simulink model "SalientPolePMSM"  (R2020b)
settings: Solver=VariableStepAuto  StartTime=0  StopTime=1  MaxStep=1e-4  RelTol=1e-4
values from neighbouring files (symbols this model uses):
  Bgain = 1    [DataSalientPolePMSM-DESKTOP-IINSHMA.m]    (also in DataSalientPolePMSM.m)
  Gcc_1ord = 1/(s/bandwidth(Gcc) + 1)    [DataSalientPolePMSM-DESKTOP-IINSHMA.m]    (also in DataSalientPolePMSM.m)
  lamdVec = mot.Ld*idVec+mot.lammg    [DataSalientPolePMSM-DESKTOP-IINSHMA.m]    (also in DataSalientPolePMSM.m)
  lamqVec = mot.Lq*iqVec    [DataSalientPolePMSM-DESKTOP-IINSHMA.m]    (also in DataSalientPolePMSM.m)
  TAB0_abc = Tabc_AB0^-1    [DataSalientPolePMSM-DESKTOP-IINSHMA.m]    (also in DataSalientPolePMSM.m)
  Tabc_AB0 = 2/3.*[     1       -1/2       -1/2 ... (first row only)    [DataSalientPolePMSM-DESKTOP-IINSHMA.m]    (also in DataSalientPolePMSM.m)
  Talphabeta_abc = Tabc_alphabeta^(-1)    [DataSalientPolePMSM-DESKTOP-IINSHMA.m]    (also in DataSalientPolePMSM.m)
undefined symbols (not defined in the file or in its folder): DiscIntNeverNeededParam, dqpll, inv, kid, kpd, magnitude, meas, mot, Obs, PI, stconv
libraries: simulink x53, pid_lib x3, powerlib x2, eeBldcCommutationLogic x1, electricdrivelib x1
(part 1 of 7)
settings Model: Creator=checc  LastModifiedBy=giuli
settings DataIOCC: SaveFormat=StructureWithTime

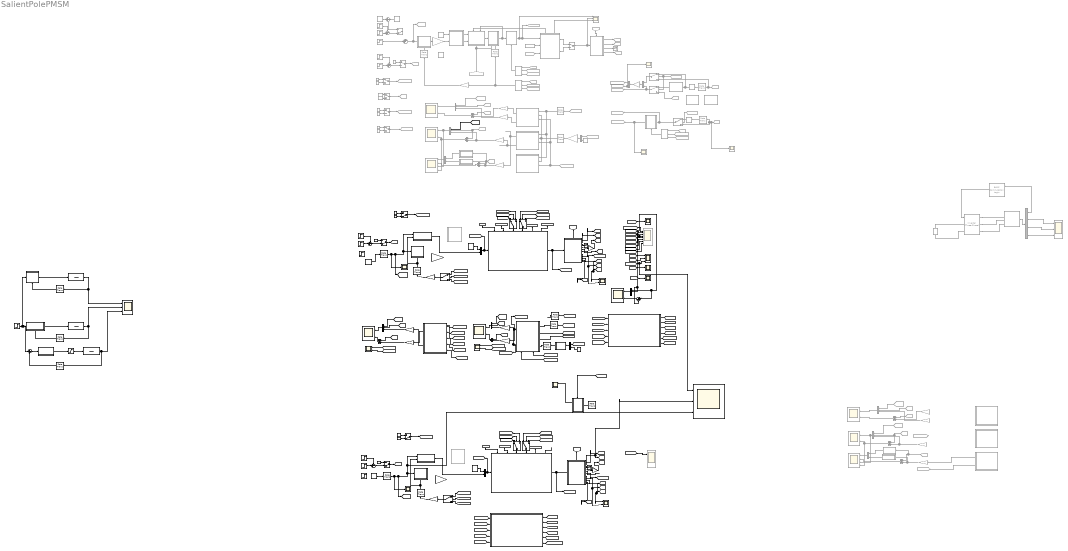
== system SalientPolePMSM ==
  note: Fuzzy Test
  note: COMMANDS
  note: GIULIO SAVIAN MODEL
  note: RICCARDO CHECHIN MODEL
  note: SIMSCAPE MODEL
  note: FEEDBACK
  note: PMSM MOTOR
  note: FIELD ORIENTED CONTROL ALGORITHM
  note: SCOPE
  note: CONTROL PANEL
  note: SENSORLESS ALGORITHM
  note: MTPA strategy
  note: FEEDBACK CHAIN
  note: INPUTS
  note: Consider the inverter
      | nonidealities or not
  note: INPUTS
  note: OUTPUTS
  note: MTPA strategy
  note: SENSORLESS ALGORITHM alpha beta axis
  note: SENSORLESS ALGORITHM dq axis (NON FUNZIONANTE)
  note: COMMANDS
  note: INPUTS
  note: FIELD ORIENTED CONTROL ALGORITHM
  note: MTPA strategy
  note: PMSM MOTOR
  " 1" : MATLAB Function  TreatAsAtomicUnit=on
  AC Voltage Source : powerlib/Electrical Sources/AC Voltage Source  Commented=on  Amplitude=100  Phase=0  Frequency=60  SampleTime=0  Measurements=None  BusType=swing  Pref=10e3  Qref=0  Qmin=-inf  Qmax=+inf
  Avarage Derivative : MATLAB Function  Commented=on  TreatAsAtomicUnit=on
  BLDC Commutation Logic : eeBldcCommutationLogic/BLDC Commutation Logic  Commented=on  Ts=-1
      settings: SourceProductBaseCode=PS
  Clarke + Park 5 : Subsystem
      settings: PortSchema="{\"entries\":[{\"content\":{\"sides\":[{\"content\":{\"connectorIds\":[\"In1\"]},\"type\":\"ConnectorPlacement.EquallySpacedRectSide\",\"uuid\":\"e456cd5a-7662-4e0b-a6c7-27ed01a0cde8\"},{\"content\":{\"connectorIds\":[\"Out1\",\"Out2\"],\"side\":\"RIGHT\"},\"type\":\"ConnectorPlacement.EquallySpacedRectSide\",\"uuid\":\"028e266b-db3d-4fa0-9acb-55f4e679375c\"},{\"content\":{\"connectorIds\":[],\"side\":\"TOP\"},\"type\":\"ConnectorPlacement.EquallySpacedRectSide\",\"uuid\":\"fc8407b0-ab5c-4984-8f89-848ec890a8d5\"},{\"content\":{\"connectorIds\":[\"In2\"],\"side\":\"BOTTOM\"},\"type\":\"ConnectorPlacement.EquallySpacedRectSide\",\"uuid\":\"5b71beec-2170-4cb0-81b8-756f92b052d7\"},{\"content\":{\"connectorIds\":[],\"side\":\"HIDDEN\"},\"type\":\"ConnectorPlacement.EquallySpacedRectSide\",\"uuid\":\"110705d2-59f3-422e-b935-78b651f69ef1\"}]},\"type\":\"ConnectorPlacement.EquallySpacedConnector\",\"uuid\":\"4a76e66d-c848-4e9c-8e50-4d720647e920\"}],\"packageUris\":[\"http://schema.mathworks.com/mf0/Connector/R2020b\"],\"version\":\"1.0\"}"
  Constant{,7,9,13} (4 alike) : Constant  Commented=on
  Constant{1,3,8,10..11} (5 alike) : Constant  Commented=on  Value=0
  Constant{5..6,12,14..15,17,21} (7 alike) : Constant  Value=0
  Constant16 : Constant
  Constant2 : Constant  Commented=on  Value=2
  Constant22 : Constant
  Constant4 : Constant  Commented=on  Value=inv.Ubus
  Control 0- Sensorless 1-Sensor : ManualSwitch  CurrentSetting=0
  Control 0- Sensorless 1-Sensor1 : ManualSwitch  CurrentSetting=0
  DER+IIR_Butterworth : MATLAB Function  Commented=on  TreatAsAtomicUnit=on
  DT SENSORLESS ALGORITHM AB : Subsystem
  DT SENSORLESS ALGORITHM DQ : Subsystem
      settings: PortSchema="{\"entries\":[{\"content\":{\"sides\":[{\"content\":{\"connectorIds\":[\"In1\",\"In2\",\"In3\",\"In4\"]},\"type\":\"ConnectorPlacement.EquallySpacedRectSide\",\"uuid\":\"b3c8a319-13c6-48fe-86bb-1433f6356212\"},{\"content\":{\"connectorIds\":[\"Out1\",\"Out2\"],\"side\":\"RIGHT\"},\"type\":\"ConnectorPlacement.EquallySpacedRectSide\",\"uuid\":\"9e7987ae-9f82-46ba-9b9e-b4e3c3a64e56\"},{\"content\":{\"connectorIds\":[],\"side\":\"TOP\"},\"type\":\"ConnectorPlacement.EquallySpacedRectSide\",\"uuid\":\"daf6aa39-0b26-4777-9886-9f84f51f9a28\"},{\"content\":{\"connectorIds\":[\"In5\",\"In6\"],\"side\":\"BOTTOM\"},\"type\":\"ConnectorPlacement.EquallySpacedRectSide\",\"uuid\":\"08005c1e-9a10-4744-b3a8-492e89e20f7c\"},{\"content\":{\"connectorIds\":[],\"side\":\"HIDDEN\"},\"type\":\"ConnectorPlacement.EquallySpacedRectSide\",\"uuid\":\"78ab3349-e4d4-4e96-9309-6e60ebf678be\"}]},\"type\":\"ConnectorPlacement.EquallySpacedConnector\",\"uuid\":\"6a0093e8-1b7a-497c-85fe-0bb07724db39\"}],\"packageUris\":[\"http://schema.mathworks.com/mf0/Connector/R2020b\"],\"version\":\"1.0\"}"
  Decoupling : Subsystem  Commented=on
      settings: PortSchema="{\"entries\":[{\"content\":{\"sides\":[{\"content\":{\"connectorIds\":[\"In1\"]},\"type\":\"ConnectorPlacement.EquallySpacedRectSide\",\"uuid\":\"366d4760-99ea-4839-93ce-cd028ffff2ed\"},{\"content\":{\"connectorIds\":[\"Out1\"],\"side\":\"RIGHT\"},\"type\":\"ConnectorPlacement.EquallySpacedRectSide\",\"uuid\":\"ffb80cd0-5569-4ccd-9b8e-dc37fbe2d6f7\"},{\"content\":{\"connectorIds\":[],\"side\":\"TOP\"},\"type\":\"ConnectorPlacement.EquallySpacedRectSide\",\"uuid\":\"2e02478e-0c74-4c41-9c3e-8c0e6bb6923b\"},{\"content\":{\"connectorIds\":[\"In2\",\"In3\"],\"side\":\"BOTTOM\"},\"type\":\"ConnectorPlacement.EquallySpacedRectSide\",\"uuid\":\"0c356034-c9d0-432b-942d-38470146113e\"}]},\"type\":\"ConnectorPlacement.EquallySpacedConnector\",\"uuid\":\"999d36d2-be3d-4c0f-9dc8-4c30e8aa3320\"}],\"packageUris\":[\"http://schema.mathworks.com/mf0/Connector/19700101\"],\"version\":\"1.0\"}"
  Demux : Demux  Commented=on  Outputs=2
  Demux1 : Demux  Commented=on
  Discrete SS ALGORITHM : Subsystem  Commented=on
  Discrete SS ALGORITHM1 : Subsystem  Commented=on
  FEEDBACK1 : Scope  Commented=on  NumInputPorts=8
  FEEDBACK2 : Scope  Commented=on  NumInputPorts=8
  FOC1 : Subsystem
      settings: PortSchema="{\"entries\":[{\"content\":{\"sides\":[{\"content\":{\"connectorIds\":[\"In1\"]},\"type\":\"ConnectorPlacement.EquallySpacedRectSide\",\"uuid\":\"8f808d96-7d84-4ca2-a92f-a817aa87351b\"},{\"content\":{\"connectorIds\":[\"Out1\"],\"side\":\"RIGHT\"},\"type\":\"ConnectorPlacement.EquallySpacedRectSide\",\"uuid\":\"5a731029-8147-494c-b637-5944669b2a42\"},{\"content\":{\"connectorIds\":[\"In2\",\"In3\",\"In4\",\"In5\",\"Out2\",\"Out3\"],\"side\":\"TOP\"},\"type\":\"ConnectorPlacement.EquallySpacedRectSide\",\"uuid\":\"612a65e4-5a0a-4716-ba74-ea18628a9a43\"},{\"content\":{\"connectorIds\":[],\"side\":\"HIDDEN\"},\"type\":\"ConnectorPlacement.EquallySpacedRectSide\",\"uuid\":\"5c37c74d-a0a6-4de5-9c93-6ea2c3953579\"}]},\"type\":\"ConnectorPlacement.EquallySpacedConnector\",\"uuid\":\"f471e1e3-c38d-4067-8334-0ee03542d9ee\"}],\"packageUris\":[\"http://schema.mathworks.com/mf0/Connector/R2020b\"],\"version\":\"1.0\"}"
  FOC2 : Subsystem
      settings: PortSchema="{\"entries\":[{\"content\":{\"sides\":[{\"content\":{\"connectorIds\":[\"In1\"]},\"type\":\"ConnectorPlacement.EquallySpacedRectSide\",\"uuid\":\"8f808d96-7d84-4ca2-a92f-a817aa87351b\"},{\"content\":{\"connectorIds\":[\"Out1\"],\"side\":\"RIGHT\"},\"type\":\"ConnectorPlacement.EquallySpacedRectSide\",\"uuid\":\"5a731029-8147-494c-b637-5944669b2a42\"},{\"content\":{\"connectorIds\":[\"In2\",\"In3\",\"In4\",\"In5\",\"Out2\",\"Out3\"],\"side\":\"TOP\"},\"type\":\"ConnectorPlacement.EquallySpacedRectSide\",\"uuid\":\"612a65e4-5a0a-4716-ba74-ea18628a9a43\"},{\"content\":{\"connectorIds\":[],\"side\":\"HIDDEN\"},\"type\":\"ConnectorPlacement.EquallySpacedRectSide\",\"uuid\":\"5c37c74d-a0a6-4de5-9c93-6ea2c3953579\"}]},\"type\":\"ConnectorPlacement.EquallySpacedConnector\",\"uuid\":\"f471e1e3-c38d-4067-8334-0ee03542d9ee\"}],\"packageUris\":[\"http://schema.mathworks.com/mf0/Connector/R2020b\"],\"version\":\"1.0\"}"
  FOC_out1 : Scope
  FeedBack: 1-MEASURE 2-SENSORLESS : ManualSwitch  Commented=on
  Feedback1 : Subsystem
  Feedback2 : Subsystem
  From : From  Commented=on  GotoTag=IABC
  From1 : From  Commented=on  GotoTag=THME_MEAS
  From10 : From  Commented=on  GotoTag=TAUL
  From{11,13,27..28,35} (5 alike) : From  Commented=on  GotoTag=THM
  From{5,14,25,29,33} (5 alike) : From  Commented=on  GotoTag=WM
  From15 : From  Commented=on  GotoTag=ON_MEAS
  From16 : From  Commented=on  GotoTag=ON_APPROX
  From17 : From  Commented=on  GotoTag=FEED
  From18 : From  Commented=on  GotoTag=WME_MEAS
  From19 : From  Commented=on  GotoTag=FEED
  From20 : From  Commented=on  GotoTag=WME_EST
  From21 : From  Commented=on  GotoTag=THME_MEAS
  From22 : From  Commented=on  GotoTag=FEED
  From23 : From  Commented=on  GotoTag=THME_EST
  From26 : From  Commented=on  GotoTag=W_REF
  From3 : From  Commented=on  GotoTag=IDQ_MEAS
  From31 : From  Commented=on  GotoTag=W_REF
  From34 : From  Commented=on  GotoTag=W_REF
  From4 : From  Commented=on  GotoTag=IABC
  From6 : From  Commented=on  GotoTag=UAB_REF
  From7 : From  Commented=on  GotoTag=THME_EST
  From8 : From  Commented=on  GotoTag=ON_MEAS
  From9 : From  Commented=on  GotoTag=IABC_MEAS
  Fuzzy PI : Subsystem
  Fuzzy PI1 : Subsystem
      settings: PortSchema="{\"entries\":[{\"content\":{\"sides\":[{\"content\":{\"connectorIds\":[\"In1\"]},\"type\":\"ConnectorPlacement.EquallySpacedRectSide\",\"uuid\":\"97881aea-ae0e-45c3-b7bb-3f05d1abc06d\"},{\"content\":{\"connectorIds\":[\"Out1\"],\"side\":\"RIGHT\"},\"type\":\"ConnectorPlacement.EquallySpacedRectSide\",\"uuid\":\"622239dd-e339-479b-bebf-0984d9e159b9\"},{\"content\":{\"connectorIds\":[],\"side\":\"TOP\"},\"type\":\"ConnectorPlacement.EquallySpacedRectSide\",\"uuid\":\"04f8ad64-72f6-4003-b853-88924601f787\"},{\"content\":{\"connectorIds\":[\"In2\"],\"side\":\"BOTTOM\"},\"type\":\"ConnectorPlacement.EquallySpacedRectSide\",\"uuid\":\"da7a61ed-22a9-4131-8461-57923f50db6b\"},{\"content\":{\"connectorIds\":[],\"side\":\"HIDDEN\"},\"type\":\"ConnectorPlacement.EquallySpacedRectSide\",\"uuid\":\"98b26063-fb72-4532-826e-e0a43804adb7\"}]},\"type\":\"ConnectorPlacement.EquallySpacedConnector\",\"uuid\":\"af8a33e1-8440-4bbf-a2b8-49fd6263fc38\"}],\"packageUris\":[\"http://schema.mathworks.com/mf0/Connector/R2020b\"],\"version\":\"1.0\"}"
  Fuzzy PI2 : Subsystem
  Gain : Gain  Commented=on  Gain=1/mot.kTau
  Gain{1,3..5,7,11..14} (9 alike) : Gain  Commented=on  Gain=1/mot.p
  Gain10 : Gain  Gain=Bgain
  Gain15 : Gain  Gain=Bgain
  Gain{9,16..17,19..21} (6 alike) : Gain  Gain=1/mot.p
  Gain18 : Gain  Gain=1/mot.kTau
  Gain2 : Gain  Commented=on  Gain=mot.p
  Gain6 : Gain  Gain=1/mot.kTau
  Gain8 : Gain  Commented=on  Gain=TAB0_abc  Multiplication=Matrix(K*u) (u vector)
  Goto : Goto  Commented=on  GotoTag=IABC
  Goto1 : Goto  Commented=on  GotoTag=THM
  Goto10 : Goto  Commented=on  GotoTag=WM
  Goto11 : Goto  Commented=on  GotoTag=FEED
  Goto12 : Goto  Commented=on  GotoTag=ON_MEAS
  Goto13 : Goto  Commented=on  GotoTag=IABC_MEAS
  Goto14 : Goto  Commented=on  GotoTag=ON_APPROX
  Goto15 : Goto  Commented=on  GotoTag=ADD_INT
  Goto16 : Goto  Commented=on  GotoTag=W_REF
  Goto18 : Goto  Commented=on  GotoTag=THME_EST
  Goto19 : Goto  Commented=on  GotoTag=WME_EST
  Goto2 : Goto  Commented=on  GotoTag=UAB_REF
  Goto3 : Goto  Commented=on  GotoTag=IDQ_MEAS
  Goto5 : Goto  Commented=on  GotoTag=WM_MEAS
  Goto6 : Goto  Commented=on  GotoTag=TAUL
  Goto7 : Goto  Commented=on  GotoTag=THME_MEAS
  Goto8 : Goto  Commented=on  GotoTag=WME_MEAS
  HPF FIR : MATLAB Function  Commented=on  TreatAsAtomicUnit=on
  INPUTS1 : Scope
  INVERTER : Subsystem  Commented=on
      settings: PortSchema="{\"entries\":[{\"content\":{\"sides\":[{\"content\":{\"connectorIds\":[\"In1\",\"In2\",\"In3\"]},\"type\":\"ConnectorPlacement.EquallySpacedRectSide\",\"uuid\":\"79c77d12-022f-42ce-98d0-f3ead9d04a95\"},{\"content\":{\"connectorIds\":[\"Out1\",\"Out2\"],\"side\":\"RIGHT\"},\"type\":\"ConnectorPlacement.EquallySpacedRectSide\",\"uuid\":\"afd498dc-a72a-45ee-96a4-44488bf591ce\"},{\"content\":{\"connectorIds\":[\"Out3\",\"Out4\"],\"side\":\"TOP\"},\"type\":\"ConnectorPlacement.EquallySpacedRectSide\",\"uuid\":\"f8f8ad46-d0da-4286-941c-855cc15ed51d\"}]},\"type\":\"ConnectorPlacement.EquallySpacedConnector\",\"uuid\":\"436ef73d-4718-409e-82fb-57ff2ccd93cf\"}],\"packageUris\":[\"http://schema.mathworks.com/mf0/Connector/R2020b\"],\"version\":\"1.0\"}"
  Inverter (Three-Phase) : electricdrivelib/Fundamental Drive Blocks/Inverter (Three-Phase)  Commented=on  LabelModeActiveChoice=Detailed  detailLevel=Detailed  driveType=Field-oriented control  Ts=2e-6  SnubberResistance=10e3  SnubberCapacitance=inf  Device=IGBT / Diodes  Ron=1e-3  ForwardVoltages=[1.2,1.2]  GTOparameters=[1e-6,2e-6]  IGBTparameters=[1e-6,2e-6]  Measurements=All voltages and currents  converterType=Inverter  SourceFrequency=60  ReferenceFrame=Rotor  dqInductances=[8.5e-3,8.5e-3]  Inductance=8.5e-3  Ls=0  Resistance=0.2  Flux=0.175  Stator_sm=[2.01e-3,4.289e-4,4.477e-3,1.354e-3]  Stator_im=[14.85e-3,0.3027e-3]  Rotor=[9.295e-3,0.3027e-3]  Lm=10.46e-3  p=4
      settings: AttributesFormatString=%<BlockChoice>  SourceProductBaseCode=PS
  MATLAB Function : MATLAB Function  Commented=on  TreatAsAtomicUnit=on
  MATLAB Function1 : MATLAB Function  Commented=on  TreatAsAtomicUnit=on
  MATLAB Function2 : MATLAB Function  Commented=on  TreatAsAtomicUnit=on
  MATLAB Function3 : MATLAB Function  Commented=on  TreatAsAtomicUnit=on
  MATLAB Function4 : MATLAB Function  Commented=on  TreatAsAtomicUnit=on
  MATLAB Function5 : MATLAB Function  Commented=on  TreatAsAtomicUnit=on
  MATLAB Function6 : MATLAB Function  Commented=on  TreatAsAtomicUnit=on
  MOTOR2 : Scope  NumInputPorts=3
  MTPA 1- id=0 0- id!=0 : Constant  Commented=on  Value=0  SampleTime=PI.vel.Ts
  MTPA 1- id=0 0- id!=1 : Constant  Commented=on  Value=0.5  SampleTime=PI.vel.Ts
  Manual Switch : ManualSwitch  Commented=on
  Measures: 0-Ideal 1-Real : ManualSwitch  Commented=on
  Multiport Switch1 : MultiPortSwitch  Commented=on  Inputs=2
  Multiport Switch2 : MultiPortSwitch  Commented=on  Inputs=2
  Multiport Switch4 : MultiPortSwitch  Commented=on  Inputs=2
  Mux{,2,4,9} (4 alike) : Mux  Commented=on  Inputs=2
  Mux1 : Mux  Inputs=2
  Mux{3,5,8,10} (4 alike) : Mux  Commented=on  Inputs=3
  Mux11 : Mux  Inputs=3
  Mux12 : Mux  Inputs=3
  Mux13 : Mux  Inputs=3
  Mux6 : Mux  Inputs=2
  Mux7 : Mux  Inputs=2
  PI_curr : Subsystem  Commented=on
      settings: PortSchema="{\"entries\":[{\"content\":{\"sides\":[{\"content\":{\"connectorIds\":[\"In1\",\"In2\"]},\"type\":\"ConnectorPlacement.EquallySpacedRectSide\",\"uuid\":\"366d4760-99ea-4839-93ce-cd028ffff2ed\"},{\"content\":{\"connectorIds\":[\"Out1\"],\"side\":\"RIGHT\"},\"type\":\"ConnectorPlacement.EquallySpacedRectSide\",\"uuid\":\"ffb80cd0-5569-4ccd-9b8e-dc37fbe2d6f7\"},{\"content\":{\"connectorIds\":[\"In3\",\"In4\"],\"side\":\"TOP\"},\"type\":\"ConnectorPlacement.EquallySpacedRectSide\",\"uuid\":\"2e02478e-0c74-4c41-9c3e-8c0e6bb6923b\"},{\"content\":{\"connectorIds\":[\"In5\"],\"side\":\"BOTTOM\"},\"type\":\"ConnectorPlacement.EquallySpacedRectSide\",\"uuid\":\"f2f25d95-a140-4291-ad57-573bdd6b43a2\"}]},\"type\":\"ConnectorPlacement.EquallySpacedConnector\",\"uuid\":\"999d36d2-be3d-4c0f-9dc8-4c30e8aa3320\"}],\"packageUris\":[\"http://schema.mathworks.com/mf0/Connector/R2020b\"],\"version\":\"1.0\"}"
  PI_i1 : Scope
  PI_i2 : Scope  NumInputPorts=2
  PI_i4 : Scope  NumInputPorts=2
  PI_speed : Subsystem  Commented=on
      settings: PortSchema="{\"entries\":[{\"content\":{\"sides\":[{\"content\":{\"connectorIds\":[\"In1\"]},\"type\":\"ConnectorPlacement.EquallySpacedRectSide\",\"uuid\":\"d6fb88a2-c1fa-4a92-9fc0-95b4e133c6fd\"},{\"content\":{\"connectorIds\":[\"Out1\"],\"side\":\"RIGHT\"},\"type\":\"ConnectorPlacement.EquallySpacedRectSide\",\"uuid\":\"95988ac3-2782-4ac1-ab79-15dc3aa515b7\"},{\"content\":{\"connectorIds\":[],\"side\":\"TOP\"},\"type\":\"ConnectorPlacement.EquallySpacedRectSide\",\"uuid\":\"6b7be8a6-9cfa-4b05-9e55-1957c44d8762\"},{\"content\":{\"connectorIds\":[\"In2\"],\"side\":\"BOTTOM\"},\"type\":\"ConnectorPlacement.EquallySpacedRectSide\",\"uuid\":\"ee05c2bf-7e6a-4cab-a0a5-16d9ad0a604f\"}]},\"type\":\"ConnectorPlacement.EquallySpacedConnector\",\"uuid\":\"554656c7-6c64-4dfa-9a52-e8b8990be749\"}],\"packageUris\":[\"http://schema.mathworks.com/mf0/Connector/19700101\"],\"version\":\"1.0\"}"
  PI_speed1 : Subsystem
      settings: PortSchema="{\"entries\":[{\"content\":{\"sides\":[{\"content\":{\"connectorIds\":[\"In1\"]},\"type\":\"ConnectorPlacement.EquallySpacedRectSide\",\"uuid\":\"d6fb88a2-c1fa-4a92-9fc0-95b4e133c6fd\"},{\"content\":{\"connectorIds\":[\"Out1\"],\"side\":\"RIGHT\"},\"type\":\"ConnectorPlacement.EquallySpacedRectSide\",\"uuid\":\"95988ac3-2782-4ac1-ab79-15dc3aa515b7\"},{\"content\":{\"connectorIds\":[],\"side\":\"TOP\"},\"type\":\"ConnectorPlacement.EquallySpacedRectSide\",\"uuid\":\"6b7be8a6-9cfa-4b05-9e55-1957c44d8762\"},{\"content\":{\"connectorIds\":[\"In2\"],\"side\":\"BOTTOM\"},\"type\":\"ConnectorPlacement.EquallySpacedRectSide\",\"uuid\":\"ee05c2bf-7e6a-4cab-a0a5-16d9ad0a604f\"}]},\"type\":\"ConnectorPlacement.EquallySpacedConnector\",\"uuid\":\"554656c7-6c64-4dfa-9a52-e8b8990be749\"}],\"packageUris\":[\"http://schema.mathworks.com/mf0/Connector/19700101\"],\"version\":\"1.0\"}"
  PI_speed2 : Subsystem
      settings: PortSchema="{\"entries\":[{\"content\":{\"sides\":[{\"content\":{\"connectorIds\":[\"In1\"]},\"type\":\"ConnectorPlacement.EquallySpacedRectSide\",\"uuid\":\"d6fb88a2-c1fa-4a92-9fc0-95b4e133c6fd\"},{\"content\":{\"connectorIds\":[\"Out1\"],\"side\":\"RIGHT\"},\"type\":\"ConnectorPlacement.EquallySpacedRectSide\",\"uuid\":\"95988ac3-2782-4ac1-ab79-15dc3aa515b7\"},{\"content\":{\"connectorIds\":[],\"side\":\"TOP\"},\"type\":\"ConnectorPlacement.EquallySpacedRectSide\",\"uuid\":\"6b7be8a6-9cfa-4b05-9e55-1957c44d8762\"},{\"content\":{\"connectorIds\":[\"In2\"],\"side\":\"BOTTOM\"},\"type\":\"ConnectorPlacement.EquallySpacedRectSide\",\"uuid\":\"ee05c2bf-7e6a-4cab-a0a5-16d9ad0a604f\"}]},\"type\":\"ConnectorPlacement.EquallySpacedConnector\",\"uuid\":\"554656c7-6c64-4dfa-9a52-e8b8990be749\"}],\"packageUris\":[\"http://schema.mathworks.com/mf0/Connector/19700101\"],\"version\":\"1.0\"}"
  PI_speed3 : Subsystem
      settings: PortSchema="{\"entries\":[{\"content\":{\"sides\":[{\"content\":{\"connectorIds\":[\"In1\"]},\"type\":\"ConnectorPlacement.EquallySpacedRectSide\",\"uuid\":\"d6fb88a2-c1fa-4a92-9fc0-95b4e133c6fd\"},{\"content\":{\"connectorIds\":[\"Out1\"],\"side\":\"RIGHT\"},\"type\":\"ConnectorPlacement.EquallySpacedRectSide\",\"uuid\":\"95988ac3-2782-4ac1-ab79-15dc3aa515b7\"},{\"content\":{\"connectorIds\":[],\"side\":\"TOP\"},\"type\":\"ConnectorPlacement.EquallySpacedRectSide\",\"uuid\":\"6b7be8a6-9cfa-4b05-9e55-1957c44d8762\"},{\"content\":{\"connectorIds\":[\"In2\"],\"side\":\"BOTTOM\"},\"type\":\"ConnectorPlacement.EquallySpacedRectSide\",\"uuid\":\"ee05c2bf-7e6a-4cab-a0a5-16d9ad0a604f\"}]},\"type\":\"ConnectorPlacement.EquallySpacedConnector\",\"uuid\":\"554656c7-6c64-4dfa-9a52-e8b8990be749\"}],\"packageUris\":[\"http://schema.mathworks.com/mf0/Connector/19700101\"],\"version\":\"1.0\"}"
  Permanent Magnet Synchronous Machine : powerlib/Machines/Permanent Magnet Synchronous Machine  Commented=on  NbPhases=3  FluxDistribution=Sinusoidal  RotorType=Round  MechanicalLoad=Torque Tm  PresetModel=No  ShowDetailedParameters=on  MeasurementBus=off  Resistance=0.0485  Inductance=8.5e-3  dqInductances=[8.5e-3,8.5e-3]  La=0.000395  MachineConstant=Flux linkage established by magnets (V.s)  Flux=0.1194  VoltageCst=86.6271  TorqueCst=0.7164  Flat=120  Mechanical=[0.0027 0.0004924 4 0]  PolePairs=4  InitialConditions=[0,0, 0,0]  InitialConditions5ph=[0 0 0 0 0 0]  RefAngle=90 degrees behind phase A axis (modified Park)  IterativeDiscreteModel=Trapezoidal non iterative  TsBlock=-1  TsPowergui=0
  Position estimation: 0-No approximation 1-With approximation : ManualSwitch  Commented=on
  Quantizer : Quantizer  Commented=on  QuantizationInterval=meas.enc.q
  Quantizer1 : Quantizer  Commented=on  QuantizationInterval=meas.cur.adc.q
  Ramp : simulink/Sources/Ramp  Commented=on  slope=(mot.WN*2*pi/60*0.7)/0.2  start=1  InitialOutput=0
  Ramp1 : simulink/Sources/Ramp  Commented=on  slope=(mot.WN*2*pi/60*0.7)/0.2  start=1.2  InitialOutput=0
  Rate Transition : RateTransition  Commented=on  OutPortSampleTime=PI.vel.Ts
  Rate Transition1 : RateTransition  Commented=on  OutPortSampleTime=meas.enc.Ts
  Rate Transition10 : RateTransition  OutPortSampleTime=100e-6
  Rate Transition{6,9,11..14,16} (7 alike) : RateTransition  OutPortSampleTime=PI.vel.Ts
  Rate Transition15 : RateTransition
  Rate Transition2 : RateTransition  Commented=on  OutPortSampleTime=inv.Tpwm
  Rate Transition3 : RateTransition  Commented=on  OutPortSampleTime=PI.cur.Ts
  Rate Transition4 : RateTransition  Commented=on  OutPortSampleTime=100e-6
  Rate Transition5 : RateTransition  Commented=on  OutPortSampleTime=100e-6
  Rate Transition7 : RateTransition  OutPortSampleTime=100e-6
  Rate Transition8 : RateTransition  OutPortSampleTime=100e-6
  Reference current : Step  Time=0  After=100  SampleTime=1/1000
  Reference current1 : Step  Time=0  After=100  SampleTime=1/1000
  Reference current2 : Step  Time=0  SampleTime=1/1000
  Repeating Sequence Stair : simulink/Sources/Repeating Sequence Stair  OutValues=[157 157 104.67 136.067 136.067 136.067 136.067 136.067].'  tsamp=1/10  OutMin=[]  OutMax=[]  OutDataTypeStr=double  OutputDataTypeScalingMode=double  OutDataType=fixdt(0,8)  ConRadixGroup=Best Precision: Vector-wise  OutScaling=2^-12
  Repeating Sequence Stair1 : simulink/Sources/Repeating Sequence Stair  OutValues=[157 157 104.67 104.67 136.067 136.067 136.067 136.067 136.067].'  tsamp=1/10  OutMin=[]  OutMax=[]  OutDataTypeStr=double  OutputDataTypeScalingMode=double  OutDataType=fixdt(0,8)  ConRadixGroup=Best Precision: Vector-wise  OutScaling=2^-12
  SENSORLESS : MATLAB Function  Commented=on  TreatAsAtomicUnit=on
  SENSORLESS ALGORITHM : Subsystem  Commented=on
  SENSORLESS ALGORITHM1 : Subsystem  Commented=on
  SENSORLESS1 : MATLAB Function  Commented=on  TreatAsAtomicUnit=on
  Saturation : Saturate  UpperLimit=10  LowerLimit=-10
  Scope : Scope  Commented=on  NumInputPorts=3
  Scope1 : Scope  Commented=on  NumInputPorts=4
  Scope{2..3,9..10} (4 alike) : Scope  Commented=on  NumInputPorts=2
  Scope11 : Scope
  Scope{12..14,16..17,20} (6 alike) : Scope  NumInputPorts=2
  Scope15 : Scope  NumInputPorts=3
  Scope18 : Scope
  Scope19 : Scope  NumInputPorts=3
  Scope4 : Scope  Commented=on
  Scope5 : Scope  Commented=on
  Scope6 : Scope  Commented=on
  Scope7 : Scope  Commented=on  NumInputPorts=4
  Scope8 : Scope  Commented=on  NumInputPorts=4
  Sensorless control: 0- simple PI 1-PI+second order integrator : ManualSwitch  Commented=on
  Step : Step  Commented=on  Time=0  After=mot.tauN*0.5  SampleTime=0
  Step1 : Step  Commented=on  Time=2  After=0.2*(mot.WN*2*pi/60)  SampleTime=PI.vel.Ts
  Step11 : Step  Time=0.6  After=mot.tauN*0.1  SampleTime=0
  Step2 : Step  Commented=on  Time=3  After=0.2*(mot.WN*2*pi/60)  SampleTime=PI.vel.Ts
  Step3 : Step  Commented=on  Time=3  After=mot.tauN*0.5  SampleTime=0
  Step4 : Step  Time=0.7  After=mot.tauN*0.1  SampleTime=0
  Step5 : Step  Time=0.6  After=mot.tauN*0.1  SampleTime=0
  Step8 : Step  Time=0.5  After=mot.tauN*0.1  SampleTime=0
  Subsystem : Subsystem
  Subsystem2 : Subsystem  Commented=on
      settings: PortSchema="{\"entries\":[{\"content\":{\"sides\":[{\"content\":{\"connectorIds\":[\"In1\"]},\"type\":\"ConnectorPlacement.EquallySpacedRectSide\",\"uuid\":\"4ed90ab9-1fa1-426e-9a51-633f86eaed93\"},{\"content\":{\"connectorIds\":[\"Out1\"],\"side\":\"RIGHT\"},\"type\":\"ConnectorPlacement.EquallySpacedRectSide\",\"uuid\":\"a783641a-eefd-4804-96bc-e093b09f1b23\"},{\"content\":{\"connectorIds\":[],\"side\":\"TOP\"},\"type\":\"ConnectorPlacement.EquallySpacedRectSide\",\"uuid\":\"b71fad55-6d7c-4fa9-b8c9-7c2d781b5980\"},{\"content\":{\"connectorIds\":[\"In2\"],\"side\":\"BOTTOM\"},\"type\":\"ConnectorPlacement.EquallySpacedRectSide\",\"uuid\":\"0ef0ee48-37c5-4f1f-a4a0-75388778f62a\"},{\"content\":{\"connectorIds\":[],\"side\":\"HIDDEN\"},\"type\":\"ConnectorPlacement.EquallySpacedRectSide\",\"uuid\":\"d9128c0c-5cc0-40ee-9c52-e819b4b0207f\"}]},\"type\":\"ConnectorPlacement.EquallySpacedConnector\",\"uuid\":\"84170b20-7cd7-4bfe-ad20-891cbad09232\"}],\"packageUris\":[\"http://schema.mathworks.com/mf0/Connector/R2020b\"],\"version\":\"1.0\"}"
  Subsystem3 : Subsystem  Commented=on
      settings: PortSchema="{\"entries\":[{\"content\":{\"sides\":[{\"content\":{\"connectorIds\":[\"In1\"]},\"type\":\"ConnectorPlacement.EquallySpacedRectSide\",\"uuid\":\"ea71606c-027e-481e-aba4-13f62585a677\"},{\"content\":{\"connectorIds\":[\"Out1\"],\"side\":\"RIGHT\"},\"type\":\"ConnectorPlacement.EquallySpacedRectSide\",\"uuid\":\"049929a5-aa1b-4856-95c9-17d9e38685d8\"},{\"content\":{\"connectorIds\":[],\"side\":\"TOP\"},\"type\":\"ConnectorPlacement.EquallySpacedRectSide\",\"uuid\":\"6c7bede6-8f52-43d3-8925-2a8f1f9ce837\"},{\"content\":{\"connectorIds\":[\"In2\"],\"side\":\"BOTTOM\"},\"type\":\"ConnectorPlacement.EquallySpacedRectSide\",\"uuid\":\"34422c14-5aba-4255-be55-6ec9502f5391\"},{\"content\":{\"connectorIds\":[],\"side\":\"HIDDEN\"},\"type\":\"ConnectorPlacement.EquallySpacedRectSide\",\"uuid\":\"23931446-a8a1-432e-a504-22fe56898a45\"}]},\"type\":\"ConnectorPlacement.EquallySpacedConnector\",\"uuid\":\"f447a990-15af-42ca-9219-73ae62b099f5\"}],\"packageUris\":[\"http://schema.mathworks.com/mf0/Connector/R2020b\"],\"version\":\"1.0\"}"
  Subtract{1..6} (6 alike) : Sum  Commented=on  Inputs=+-
  Subtract7 : Sum  Inputs=+-
  Subtract8 : Sum  Inputs=+-
  Sum : Sum  Commented=on  Inputs=++|
  Sum1 : Sum  Commented=on  Inputs=-+|
  Sum10 : Sum  Inputs=-+|
  Sum2 : Sum  Commented=on  Inputs=-+|
  Sum3 : Sum  Commented=on  Inputs=+|-
  Sum4 : Sum  Inputs=|+-
  Sum5 : Sum  Inputs=-+|
  Sum6 : Sum  Inputs=|+-
  Switch : Switch  Commented=on  Criteria=u2 > Threshold
  Switch{1..2,5..8} (6 alike) : Switch  Criteria=u2 > Threshold
  Switch3 : Switch  Commented=on  Criteria=u2 > Threshold
  Switch4 : Switch  Commented=on  Criteria=u2 > Threshold
  Synchronous motor1 : Subsystem
      settings: PortSchema="{\"entries\":[{\"content\":{\"sides\":[{\"content\":{\"connectorIds\":[\"In1\"]},\"type\":\"ConnectorPlacement.EquallySpacedRectSide\",\"uuid\":\"48717f00-8aab-421a-92ef-39631ca05127\"},{\"content\":{\"connectorIds\":[\"Out1\",\"Out2\",\"Out3\",\"Out4\",\"Out5\",\"Out6\",\"Out7\",\"Out8\",\"Out9\",\"Out10\"],\"side\":\"RIGHT\"},\"type\":\"ConnectorPlacement.EquallySpacedRectSide\",\"uuid\":\"5a0867b8-e422-4f84-89ea-5ba0ff3dbf16\"},{\"content\":{\"connectorIds\":[\"In2\"],\"side\":\"TOP\"},\"type\":\"ConnectorPlacement.EquallySpacedRectSide\",\"uuid\":\"701177a4-a309-4311-81d1-a6e4439a5b4a\"}]},\"type\":\"ConnectorPlacement.EquallySpacedConnector\",\"uuid\":\"5c7a4b9e-8ad2-47b2-9a58-fcbb5c2072f8\"}],\"packageUris\":[\"http://schema.mathworks.com/mf0/Connector/R2020b\"],\"version\":\"1.0\"}"
  Synchronous motor2 : Subsystem  Commented=on
      settings: PortSchema="{\"entries\":[{\"content\":{\"sides\":[{\"content\":{\"connectorIds\":[\"In1\"]},\"type\":\"ConnectorPlacement.EquallySpacedRectSide\",\"uuid\":\"48717f00-8aab-421a-92ef-39631ca05127\"},{\"content\":{\"connectorIds\":[\"Out1\",\"Out2\",\"Out3\",\"Out4\"],\"side\":\"RIGHT\"},\"type\":\"ConnectorPlacement.EquallySpacedRectSide\",\"uuid\":\"5a0867b8-e422-4f84-89ea-5ba0ff3dbf16\"},{\"content\":{\"connectorIds\":[\"In2\"],\"side\":\"TOP\"},\"type\":\"ConnectorPlacement.EquallySpacedRectSide\",\"uuid\":\"701177a4-a309-4311-81d1-a6e4439a5b4a\"}]},\"type\":\"ConnectorPlacement.EquallySpacedConnector\",\"uuid\":\"5c7a4b9e-8ad2-47b2-9a58-fcbb5c2072f8\"}],\"packageUris\":[\"http://schema.mathworks.com/mf0/Connector/19700101\"],\"version\":\"1.0\"}"
  Synchronous motor3 : Subsystem
      settings: PortSchema="{\"entries\":[{\"content\":{\"sides\":[{\"content\":{\"connectorIds\":[\"In1\"]},\"type\":\"ConnectorPlacement.EquallySpacedRectSide\",\"uuid\":\"48717f00-8aab-421a-92ef-39631ca05127\"},{\"content\":{\"connectorIds\":[\"Out1\",\"Out2\",\"Out3\",\"Out4\",\"Out5\",\"Out6\",\"Out7\",\"Out8\",\"Out9\",\"Out10\"],\"side\":\"RIGHT\"},\"type\":\"ConnectorPlacement.EquallySpacedRectSide\",\"uuid\":\"5a0867b8-e422-4f84-89ea-5ba0ff3dbf16\"},{\"content\":{\"connectorIds\":[\"In2\"],\"side\":\"TOP\"},\"type\":\"ConnectorPlacement.EquallySpacedRectSide\",\"uuid\":\"701177a4-a309-4311-81d1-a6e4439a5b4a\"}]},\"type\":\"ConnectorPlacement.EquallySpacedConnector\",\"uuid\":\"5c7a4b9e-8ad2-47b2-9a58-fcbb5c2072f8\"}],\"packageUris\":[\"http://schema.mathworks.com/mf0/Connector/R2020b\"],\"version\":\"1.0\"}"
  Terminator : Terminator  Commented=on
  Terminator1 : Terminator
  Terminator2 : Terminator
  Transfer Fcn : TransferFcn  Denominator=[1 1]
  Transfer Fcn1 : TransferFcn  Denominator=[1 1]
  Transfer Fcn2 : TransferFcn  Denominator=[1 1]
  base speed %Wn : Step  Commented=on  Time=0  After=0.3*(mot.WN*2*pi/60)  SampleTime=PI.vel.Ts
  inserimento carico : ManualSwitch  Commented=on
  inserimento carico1 : ManualSwitch  CurrentSetting=0
  inserimento carico2 : ManualSwitch  CurrentSetting=0
  inserimento gradino di W : ManualSwitch  Commented=on  CurrentSetting=0
  wires:
  Synchronous motor2/3(taum) -> Terminator/1
  Synchronous motor2/2(wm) -> Goto10/1  "wm"
  Synchronous motor2/1(thm) -> Goto1/1
  Constant4/1 -> INVERTER/2(uBus)
  From/1 -> INVERTER/3(iabc)
  INVERTER/1(uabc_n*) -> Manual Switch/1
  INVERTER/2(uabc_n*nonideal) -> Manual Switch/2
  MATLAB Function/1(id) -> PI_curr/1(id*)  "id*"
  INVERTER/3(satON) -> PI_curr/3(satON)  "anti-windup mechanism"
  MATLAB Function/2(iq) -> PI_curr/2(iq*)
  PI_speed/1(tau*sat) -> Gain/1
  Sum2/1 -> inserimento carico/2
  Rate Transition/1 -> PI_speed/2(wm)
  From11/1 -> Switch3/3, Rate Transition1/1
  From4/1 -> Scope4/1, Switch/3, Rate Transition2/1
  Switch4/1 -> Mux/2, Goto5/1
  Mux/1 -> Gain2/1
  Gain2/1 -> Demux/1
  Demux/1 -> Goto7/1
  Subsystem2/1(dq) -> Scope5/1, Goto3/1
  Rate Transition3/1 -> Decoupling/3(wme)
  From9/1 -> Rate Transition5/1
  Rate Transition4/1 -> SENSORLESS/2(uabc), SENSORLESS ALGORITHM/2(uabc), Discrete SS ALGORITHM/2(uabc)
  From13/1 -> Subtract1/1, MATLAB Function1/1(th)
  Subtract1/1 -> Scope1/2  "ERR"
  From14/1 -> Subtract2/1, Mux3/2  "WM"
  Gain7/1 -> MATLAB Function2/1(th), Subtract1/2  "THM_EST"
  SENSORLESS ALGORITHM/1(thme_est) -> Gain1/1
  SENSORLESS ALGORITHM/2(wme_est) -> Gain4/1
  From3/1 -> Decoupling/2(idq), PI_curr/5(idq)
  FeedBack: 1-MEASURE 2-SENSORLESS/1 -> Goto11/1
  From17/1 -> Multiport Switch1/1
  From7/1 -> Multiport Switch1/3
  From1/1 -> Multiport Switch1/2
  Multiport Switch1/1 -> Subsystem3/2(thme)
  Constant/1 -> FeedBack: 1-MEASURE 2-SENSORLESS/1
  Constant2/1 -> FeedBack: 1-MEASURE 2-SENSORLESS/2
  From18/1 -> Multiport Switch2/2
  From20/1 -> Multiport Switch2/3
  From19/1 -> Multiport Switch2/1
  Multiport Switch2/1 -> Gain3/1, Rate Transition3/1
  Gain3/1 -> Rate Transition/1
  From21/1 -> Multiport Switch4/2
  From22/1 -> Multiport Switch4/1
  From23/1 -> Multiport Switch4/3
  Multiport Switch4/1 -> Subsystem2/2(thme)
  Sum/1 -> Goto16/1, PI_speed/1(wm*)
  Synchronous motor2/4(iabc) -> Goto/1
  Manual Switch/1 -> Scope7/2, Synchronous motor2/1(uabc)
  Switch/1 -> Goto13/1, Subsystem2/1(abc)
  Quantizer/1 -> Switch3/1, HPF FIR/1(thm)
  [W_REF] -> Mux3/1  "W_REF"
  Gain5/1 -> Mux3/3, Subtract2/2  "WM_EST"
  Subtract2/1 -> Scope1/4, Scope3/2  "ERR"
  Discrete SS ALGORITHM/2(wme_est) -> Gain5/1
  From16/1 -> SENSORLESS ALGORITHM/3(ON_approx), Discrete SS ALGORITHM/3(ON_approx), SENSORLESS/3(ON_approx)  "ON approx"
  Discrete SS ALGORITHM/1(thme_est) -> Gain7/1
  From6/1 -> Mux2/1
  Mux2/1 -> Gain8/1
  Constant8/1 -> Mux2/2
  Quantizer1/1 -> Switch/1
  Rate Transition2/1 -> Quantizer1/1
  From8/1 -> Switch/2
  Rate Transition1/1 -> Quantizer/1
  Switch3/1 -> Mux/1
  HPF FIR/1(wm) -> Switch4/1
  From5/1 -> Switch4/3
  From15/1 -> Switch4/2, Switch3/2
  Constant9/1 -> Measures: 0-Ideal 1-Real/2
  Constant10/1 -> Measures: 0-Ideal 1-Real/1
  Measures: 0-Ideal 1-Real/1 -> Goto12/1
  Gain8/1 -> Rate Transition4/1
  Rate Transition5/1 -> SENSORLESS/1(iabc), Discrete SS ALGORITHM/1(iabc), SENSORLESS ALGORITHM/1(iabc)
  Constant3/1 -> Position estimation: 0-No approximation 1-With approximation/1
  Constant7/1 -> Position estimation: 0-No approximation 1-With approximation/2
  Position estimation: 0-No approximation 1-With approximation/1 -> Goto14/1
  inserimento carico/1 -> Goto6/1
  Constant11/1 -> inserimento carico/1
  base speed %Wn/1 -> Sum/2
  Step1/1 -> Sum1/2
  MTPA 1- id=0 0- id!=0/1 -> MATLAB Function/1(OffMtpa)
  MATLAB Function1/1(thMod) -> Mux4/1  "THM"
  MATLAB Function2/1(thMod) -> Mux4/2  "THM_EST"
  Mux3/1 -> Scope1/3, Scope3/1
  Mux4/1 -> Scope1/1
  Step/1 -> Sum2/2
  Step3/1 -> Sum2/1
  ? -> SENSORLESS ALGORITHM/4(ADD_integrator), SENSORLESS/4(data), Discrete SS ALGORITHM/4(ADD_integrator)
  Sensorless control: 0- simple PI 1-PI+second order integrator/1 -> Goto15/1
  Constant13/1 -> Sensorless control: 0- simple PI 1-PI+second order integrator/2
  Constant1/1 -> Sensorless control: 0- simple PI 1-PI+second order integrator/1
  Mux5/1 -> Scope2/1
  Subtract3/1 -> Scope2/2  "ERR"
  Gain4/1 -> Mux5/3  "WM_EST"
  From26/1 -> Mux5/1  "W_REF"
  From25/1 -> Mux5/2  "WM"
  Sum1/1 -> inserimento gradino di W/2
  Step2/1 -> Sum1/1
  Ramp/1 -> Sum3/1
  Ramp1/1 -> Sum3/2
  Sum3/1 -> inserimento gradino di W/1
  From27/1 -> Subtract3/1
  Gain1/1 -> Subtract3/2  "THM_EST"
  From10/1 -> Synchronous motor2/2(tauL)
  Demux/2 -> Scope6/1, Goto8/1
  Synchronous motor3/4(iabc) -> Gain10/1
  Gain10/1 -> [IABC]
  [WME_MEAS] -> FEEDBACK1/2
  [THME_MEAS] -> FEEDBACK1/1
  [IABC_MEAS] -> FEEDBACK1/5
  [WM_MEAS] -> FEEDBACK1/3, Sum6/2, Mux13/2
  [IDQ_MEAS] -> FEEDBACK1/6
  [UDQ] -> PI_i1/1
  FOC1/3(UDQ) -> [UDQ]
  [IDQ_MEAS] -> FOC1/3(IDQ_MEAS)
  [IABC] -> FOC1/2(IABC)
  FOC1/2(UAB_REF) -> [UAB_REF]
  [Iq] -> INPUTS1/1
  [UABC] -> FOC_out1/1
  [IABC] -> MOTOR2/1
  [THM] -> MOTOR2/2
  [WM] -> Scope19/1, MOTOR2/3
  [THME_EST] -> Feedback1/5(THME_EST)
  [WM] -> Feedback1/4(WM)
  [ON_MEAS] -> Feedback1/3(ON_MEAS)
  Feedback1/1(THME_MEAS) -> [THME_MEAS]
  Feedback1/3(WM_MEAS) -> [WM_MEAS]
  Feedback1/4(IABC_MEAS) -> [IABC_MEAS]
  Feedback1/5(IDQ_MEAS) -> [IDQ_MEAS]
  Feedback1/2(WME_MEAS) -> [WME_MEAS]
  [THM] -> Feedback1/1(THM)
  [IABC] -> Feedback1/2(IABC)
  Synchronous motor3/2(wm) -> [WM]  "wm"
  Synchronous motor3/1(thm) -> [THM]
  Synchronous motor3/3(taum) -> Terminator2/1
  inserimento carico2/1 -> [TAUL]
  Sum10/1 -> inserimento carico2/2
  Step8/1 -> Sum10/2
  Step11/1 -> Sum10/1
  Constant14/1 -> inserimento carico2/1
  [TAUL] -> Synchronous motor3/2(tauL)
  BLDC Commutation Logic/1 -> Inverter (Three-Phase)/1
  Permanent Magnet Synchronous Machine/1 -> Demux1/1
  Demux1/1 -> BLDC Commutation Logic/1
  Demux1/2 -> Scope/1
  Demux1/3 -> Scope/2
  Demux1/4 -> Scope/3
  Subsystem3/1(AB) -> Scope7/1, INVERTER/1(uAB), Goto2/1
  INVERTER/4(duties) -> Scope7/3
  FOC1/1(uabc*) -> Synchronous motor3/1(uabc), [UABC]
  Gain/1 -> MATLAB Function/2(i_ref)
  Rate Transition6/1 -> PI_speed1/2(wm), Fuzzy PI/2(wm)
  Mux6/1 -> FOC1/1(iq*), [IDQ_REF]
  Gain9/1 -> Rate Transition6/1
  Mux9/1 -> Scope8/1
  MATLAB Function4/1(thMod) -> Mux9/1  "THM"
  From31/1 -> Mux8/1  "W_REF"
  Gain12/1 -> Mux10/3  "WM_EST"
  From33/1 -> Mux10/2  "WM"
  From34/1 -> Mux10/1  "W_REF"
  Mux8/1 -> Scope10/1, Scope8/3
  MATLAB Function5/1(thMod) -> Mux9/2  "THM_EST"
  Gain13/1 -> Mux8/3, Subtract5/2  "WM_EST"
  Gain11/1 -> Subtract6/2  "THM_EST"
  From29/1 -> Subtract5/1, Mux8/2  "WM"
  Subtract4/1 -> Scope8/2  "ERR"
  Gain14/1 -> MATLAB Function5/1(th), Subtract4/2  "THM_EST"
  From35/1 -> Subtract6/1
  From28/1 -> Subtract4/1, MATLAB Function4/1(th)
  Mux10/1 -> Scope9/1
  Subtract6/1 -> Scope9/2  "ERR"
  Subtract5/1 -> Scope8/4, Scope10/2  "ERR"
  [IABC_MEAS] -> Rate Transition8/1
  SENSORLESS1/1(thme_est) -> Gain14/1
  SENSORLESS1/2(wme_est) -> Goto19/1
  Mux11/1 -> Scope12/1
  [THM] -> Subtract7/1
  [WM] -> Mux11/2  "WM"
  Gain17/1 -> Mux11/3  "WM_EST"
  Gain16/1 -> Subtract7/2  "THM_EST"
  [W_REF] -> Mux11/1  "W_REF"
  Subtract7/1 -> Scope12/2  "ERR"
  DT SENSORLESS ALGORITHM DQ/1(thme_est) -> [THME_EST], Gain16/1
  Rate Transition8/1 -> DT SENSORLESS ALGORITHM DQ/1(iabc1)
  [THM] -> Subtract8/1
  Subtract8/1 -> Scope14/2  "ERR"
  Mux12/1 -> Scope14/1
  [WM] -> Mux12/2  "WM"
  Gain19/1 -> Subtract8/2  "THM_EST"
  [W_REF] -> Mux12/1  "W_REF"
  Gain20/1 -> Mux12/3  "WM_EST"
  [IABC_MEAS] -> DT SENSORLESS ALGORITHM AB/2(iabc)
  Constant22/1 -> Control 0- Sensorless 1-Sensor/2
  Constant21/1 -> Control 0- Sensorless 1-Sensor/1
  Control 0- Sensorless 1-Sensor/1 -> [ON_SENSOR]
  [ON_SENSOR] -> Switch1/2
  [WME_EST] -> Switch1/3
  DT SENSORLESS ALGORITHM DQ/2(wme_est) -> [WME_EST], Gain17/1
  [ON_SENSOR] -> Switch2/2
  [ON_SENSOR] -> Feedback1/6(IABC1)
  DT SENSORLESS ALGORITHM AB/2(wme_est) -> Gain20/1
  DT SENSORLESS ALGORITHM AB/1(thme_est) -> Gain19/1
  PI_curr/1(udq*) -> Decoupling/1(udq*)
  Decoupling/1(udq**) -> Subsystem3/1(dq), PI_curr/4(udq_sat)  "udq_sat  for anti-windup mechanism"
  Subsystem/1(abc) -> Rate Transition7/1
  Mux1/1 -> Subsystem/1(In1)
  [ON_SENSOR] -> Switch5/2
  [THME_EST] -> Scope17/2
  [THME_MEAS] -> Scope17/1
  [UDQ] -> FEEDBACK1/7
  [UABC] -> FEEDBACK1/8
  Synchronous motor3/5(idq) -> [IDQ]
  Synchronous motor3/7(w_me) -> [WME]
  Synchronous motor3/6(theta_me) -> [THME]
  [IDQ_MEAS] -> Rate Transition10/1
  Rate Transition10/1 -> ?
  Synchronous motor3/8(U_A) -> PI_i2/2, [UA]
  [UA] -> DT SENSORLESS ALGORITHM AB/3(UA)
  [UB] -> DT SENSORLESS ALGORITHM AB/4(UB)
  [W_REF] -> Sum6/1, Mux13/1, FEEDBACK1/4
  Reference current2/1 -> PI_speed2/1(wm*), Sum4/1, Fuzzy PI1/1(wm*)
  PI_speed2/1(tau*sat) -> Transfer Fcn/1
  Fuzzy PI1/1(tau*sat) -> Transfer Fcn1/1
  Transfer Fcn1/1 -> Scope15/2, Rate Transition12/1
  Transfer Fcn/1 -> Scope15/1, Rate Transition11/1
  Rate Transition11/1 -> PI_speed2/2(wm)
  Rate Transition12/1 -> Fuzzy PI1/2(wm)
  " 1"/1(rawoutput) -> Saturation/1
  Saturation/1 -> Transfer Fcn2/1  "tau*sat"
  Transfer Fcn2/1 -> Rate Transition13/1, Scope15/3
  Sum4/1 -> " 1"/1(err)
  Rate Transition13/1 -> Sum4/2
  [WME_MEAS] -> Switch1/1
  [THME_EST] -> Switch2/3
  [WME_MEAS] -> Switch5/1
  Switch5/1 -> FOC1/5(WME_MEAS)
  Switch1/1 -> Gain9/1
  [THME_MEAS] -> Switch2/1
  [WME_EST] -> Switch5/3
  Switch2/1 -> FOC1/4(THME_MEAS)
  [WME_MEAS] -> DT SENSORLESS ALGORITHM AB/1(wel_meas)
  [THME_MEAS] -> Scope16/1
  [THME_EST] -> Scope16/2
  Synchronous motor3/9(U_B) -> PI_i2/1, [UB]
  Rate Transition9/1 -> Scope11/1, [W_REF], Fuzzy PI/1(wm*), PI_speed1/1(wm*)
  Constant5/1 -> Mux6/1
  [UDQ] -> DT SENSORLESS ALGORITHM DQ/3(udq)
  [WME_MEAS] -> DT SENSORLESS ALGORITHM DQ/6(wme)
  Rate Transition15/1 -> Clarke + Park 5/1(abc)
  Clarke + Park 5/2(AB) -> Scope13/1
  [THM] -> Clarke + Park 5/2(thme)
  [THME_MEAS] -> DT SENSORLESS ALGORITHM DQ/5(thme1)
  Constant6/1 -> Mux1/2
  [UAB_REF] -> Mux1/1
  Rate Transition7/1 -> DT SENSORLESS ALGORITHM DQ/4(In3)
  Synchronous motor3/10(U_DQ) -> [UDQ2]
  [UDQ2] -> DT SENSORLESS ALGORITHM DQ/2(udq_est)
  [THME_MEAS] -> ?
  [UAB_REF] -> DT SENSORLESS ALGORITHM AB/5(In6)
  Repeating Sequence Stair1/1 -> Rate Transition16/1
  Control 0- Sensorless 1-Sensor1/1 -> [ON_SENSOR2]
  [WME_MEAS2] -> FEEDBACK2/2
  Constant17/1 -> Mux7/1
  Switch6/1 -> Gain21/1
  Synchronous motor1/10(U_DQ) -> [UDQ3]
  [WME_MEAS2] -> Switch8/1
  Switch7/1 -> FOC2/4(THME_MEAS)
  Synchronous motor1/8(U_A) -> PI_i4/2, [UA2]
  Rate Transition16/1 -> Scope18/1, [W_REF2], Fuzzy PI2/1(wm*), Scope19/3, PI_speed3/1(wm*)
  Constant16/1 -> Control 0- Sensorless 1-Sensor1/2
  [THME_MEAS2] -> Switch7/1
  [WME_MEAS2] -> Switch6/1
  ? -> FEEDBACK2/1
  Synchronous motor1/6(theta_me) -> [THME2]
  Synchronous motor1/7(w_me) -> [WME2]
  Synchronous motor1/5(idq) -> ?
  Constant15/1 -> Control 0- Sensorless 1-Sensor1/1
  [TAUL2] -> Synchronous motor1/2(tauL)
  [ON_SENSOR2] -> Switch7/2
  [WME_EST2] -> Switch8/3
  [ON_SENSOR2] -> Switch6/2
  Synchronous motor1/2(wm) -> Scope19/2, [WM2]  "wm"
  Step5/1 -> Sum5/2
  [ON_SENSOR2] -> Switch8/2
  Synchronous motor1/9(U_B) -> PI_i4/1, [UB2]
  Rate Transition14/1 -> PI_speed3/2(wm), Fuzzy PI2/2(wm)
  FOC2/1(uabc*) -> Synchronous motor1/1(uabc), [UABC2]
  inserimento carico1/1 -> [TAUL2]
  Synchronous motor1/1(thm) -> [THM2]
  Mux7/1 -> FOC2/1(iq*), [IDQ_REF2]
  [THME_EST2] -> Switch7/3
  Constant12/1 -> inserimento carico1/1
  FOC2/2(UAB_REF) -> [UAB_REF2]
  Step4/1 -> Sum5/1
  Sum5/1 -> inserimento carico1/2
  [WME_EST2] -> Switch6/3
  Switch8/1 -> FOC2/5(WME_MEAS)
  [IABC2] -> FOC2/2(IABC)
  FOC2/3(UDQ) -> ?
  Gain21/1 -> Rate Transition14/1
  [IDQ_MEAS2] -> FOC2/3(IDQ_MEAS)
  Synchronous motor1/4(iabc) -> Gain15/1
  Synchronous motor1/3(taum) -> Terminator1/1
  Gain15/1 -> [IABC2]
  Fuzzy PI2/1(tau*sat) -> Mux7/2
  [ON_SENSOR2] -> Feedback2/6(IABC1)
  Feedback2/1(THME_MEAS) -> [THME_MEAS2]
  Feedback2/2(WME_MEAS) -> [WME_MEAS2]
  Feedback2/3(WM_MEAS) -> [WM_MEAS2]
  [THM2] -> Feedback2/1(THM)
  [THME_EST2] -> Feedback2/5(THME_EST)
  Feedback2/4(IABC_MEAS) -> [IABC_MEAS2]
  Feedback2/5(IDQ_MEAS) -> [IDQ_MEAS2]
  [WM2] -> Feedback2/4(WM)
  [ON_MEAS2] -> Feedback2/3(ON_MEAS)
  [IABC2] -> Feedback2/2(IABC)
  Fuzzy PI/1(tau*sat) -> Mux6/2
  Mux13/1 -> Scope20/1
  Sum6/1 -> Scope20/2
  Repeating Sequence Stair/1 -> Rate Transition9/1
  connections:
  Inverter (Three-Phase)/RConn1 -- Permanent Magnet Synchronous Machine/LConn1
  Inverter (Three-Phase)/RConn2 -- Permanent Magnet Synchronous Machine/LConn2
  Inverter (Three-Phase)/RConn3 -- Permanent Magnet Synchronous Machine/LConn3
  AC Voltage Source/RConn1 -- Inverter (Three-Phase)/LConn1
  Inverter (Three-Phase)/LConn2 -- AC Voltage Source/LConn1

== system SalientPolePMSM/Clarke + Park 5 ==
  note: INPUTS
  note: OUTPUT
  note: INPUTS
  abc : Inport
  thme : Inport  Port=2
  Add1 : Sum  Inputs=+-
  Add2 : Sum
  Add3 : Sum  Inputs=-+
  Add4 : Sum
  Cos1 : Trigonometry  Operator=cos
  Cos2 : Trigonometry  Operator=cos
  Demux1 : Demux  Outputs=3
  Demux2 : Demux  Outputs=3
  Demux3 : Demux  Outputs=3
  Gain : Gain  Gain=sqrt(3)
  Gain1 : Gain  Gain=Tabc_AB0  Multiplication=Matrix(K*u) (u vector)
  Gain10 : Gain  Gain=-1/sqrt(3)
  Gain2 : Gain  Gain=1/2
  Gain9 : Gain  Gain=2
  Mux : Mux  Inputs=2
  Mux1 : Mux  Inputs=2
  Mux2 : Mux  Inputs=3
  Product{,1..7} (8 alike) : Product
  Scope : Scope  NumInputPorts=2
  Sin1 : Trigonometry
  Sin2 : Trigonometry
  Sum2 : Sum  Inputs=--|
  Sum5 : Sum  Inputs=++|
  Terminator : Terminator
  Terminator1 : Terminator
  dq : Outport
  AB : Outport  Port=2
  wires:
  Demux2/3 -> Terminator/1
  Product/1 -> Add2/1
  Product1/1 -> Add2/2
  Cos2/1 -> Product/2, Product3/1
  Demux2/1 -> Product3/2, Product1/1
  Product3/1 -> Add3/2
  Product2/1 -> Add3/1
  Demux2/2 -> Product2/1, Product/1
  Sin2/1 -> Product2/2, Product1/2
  Add3/1 -> Mux1/2
  Add2/1 -> Mux1/1
  Sum5/1 -> Gain10/1
  Gain9/1 -> Sum5/2
  Demux1/2 -> Gain9/1
  Demux1/3 -> Mux2/3
  Demux1/1 -> Mux2/1, Sum5/1
  Gain10/1 -> Mux2/2
  Gain1/1 -> AB/1, Demux2/1, Scope/1
  Add1/1 -> Mux/1
  Sin1/1 -> Product5/2, Product4/2
  Gain/1 -> Sum2/2
  Product5/1 -> Add1/2
  Cos1/1 -> Product6/2, Product7/1
  Sum2/1 -> Gain2/1
  Demux3/1 -> Product5/1, Product6/1, Sum2/1
  Demux3/2 -> Gain/1
  Product4/1 -> Add4/2
  Product7/1 -> Add1/1
  Product6/1 -> Add4/1
  Demux3/3 -> Terminator1/1
  Add4/1 -> Mux/2
  Gain2/1 -> Product7/2, Product4/1
  thme/1 -> Sin2/1, Cos2/1
  Mux1/1 -> dq/1
  abc/1 -> Gain1/1

== system SalientPolePMSM/DT SENSORLESS ALGORITHM AB ==
  wel_meas : Inport
  iabc : Inport  Port=2
  UA : Inport  Port=3
  UB : Inport  Port=4
  In6 : Inport  Port=5
  Classic PLL1 : Subsystem
      settings: PortSchema="{\"entries\":[{\"content\":{\"sides\":[{\"content\":{\"connectorIds\":[\"In1\",\"In2\"]},\"type\":\"ConnectorPlacement.EquallySpacedRectSide\",\"uuid\":\"e7ca337f-f955-4a95-8861-4994a03ba33f\"},{\"content\":{\"connectorIds\":[\"Out1\",\"Out2\"],\"side\":\"RIGHT\"},\"type\":\"ConnectorPlacement.EquallySpacedRectSide\",\"uuid\":\"be7a5401-2ea2-4b14-8c0d-fa9893fe0dc3\"},{\"content\":{\"connectorIds\":[\"In3\"],\"side\":\"TOP\"},\"type\":\"ConnectorPlacement.EquallySpacedRectSide\",\"uuid\":\"18ac00f1-60dc-4819-8439-82afdaabcc73\"},{\"content\":{\"connectorIds\":[],\"side\":\"HIDDEN\"},\"type\":\"ConnectorPlacement.EquallySpacedRectSide\",\"uuid\":\"ec78e6b1-3cd9-445e-bf6b-ea38fea55f7c\"}]},\"type\":\"ConnectorPlacement.EquallySpacedConnector\",\"uuid\":\"0d1e30ca-7d4c-4552-9b67-43c395697d8a\"}],\"packageUris\":[\"http://schema.mathworks.com/mf0/Connector/R2020b\"],\"version\":\"1.0\"}"
  Demux : Demux  Outputs=2
  Demux3 : Demux  Outputs=2
  Discrete Filter1 : DiscreteFilter  Numerator=[Obs.lpf.alpha]  Denominator=[1 ((Obs.lpf.alpha)-1)]  SampleTime=Obs.Ts
  Discrete Filter2 : DiscreteFilter  Numerator=[Obs.lpf.alpha]  Denominator=[1 (Obs.lpf.alpha-1)]  SampleTime=Obs.Ts
  Discrete Filter3 : DiscreteFilter  Numerator=[Obs.lpf.alpha/3]  Denominator=[1 ((Obs.lpf.alpha/3)-1)]  SampleTime=Obs.Ts
  Normalized and improved PLL2 : Subsystem
  Observer : Subsystem  Commented=on
  PII : Subsystem
  Rate Transition2 : RateTransition
  Rate Transition3 : RateTransition
  Rev_Park + Rev_Clarke1 : Subsystem
  Scope : Scope  NumInputPorts=2
  Scope1 : Scope  NumInputPorts=2
  Scope2 : Scope  NumInputPorts=3
  Scope3 : Scope  NumInputPorts=4
  Transfer Fcn : TransferFcn  Numerator=[inv.Ts 0]  Denominator=[inv.Ts 1]
  Transfer Fcn1 : TransferFcn  Numerator=[inv.Ts 0]  Denominator=[inv.Ts 1]
  alpha axis observer : Subsystem
      settings: PortSchema="{\"entries\":[{\"content\":{\"sides\":[{\"content\":{\"connectorIds\":[\"In1\"]},\"type\":\"ConnectorPlacement.EquallySpacedRectSide\",\"uuid\":\"b996c3cd-9b24-4489-b39b-20b2ab7fe738\"},{\"content\":{\"connectorIds\":[\"Out1\",\"Out2\"],\"side\":\"RIGHT\"},\"type\":\"ConnectorPlacement.EquallySpacedRectSide\",\"uuid\":\"c70de7f2-3715-43c3-9599-c736073893c8\"},{\"content\":{\"connectorIds\":[\"In2\",\"In3\"],\"side\":\"TOP\"},\"type\":\"ConnectorPlacement.EquallySpacedRectSide\",\"uuid\":\"1a48b6dd-1bbf-47fb-a945-4a4baa930d91\"},{\"content\":{\"connectorIds\":[],\"side\":\"HIDDEN\"},\"type\":\"ConnectorPlacement.EquallySpacedRectSide\",\"uuid\":\"709f434a-be22-4ab0-8c88-5861684d60a0\"}]},\"type\":\"ConnectorPlacement.EquallySpacedConnector\",\"uuid\":\"7491e8e9-2ed3-4647-a2c4-91fc44b544f7\"}],\"packageUris\":[\"http://schema.mathworks.com/mf0/Connector/R2020b\"],\"version\":\"1.0\"}"
  alpha axis observer2 : Subsystem
      settings: PortSchema="{\"entries\":[{\"content\":{\"sides\":[{\"content\":{\"connectorIds\":[\"In1\"]},\"type\":\"ConnectorPlacement.EquallySpacedRectSide\",\"uuid\":\"b996c3cd-9b24-4489-b39b-20b2ab7fe738\"},{\"content\":{\"connectorIds\":[\"Out1\",\"Out2\"],\"side\":\"RIGHT\"},\"type\":\"ConnectorPlacement.EquallySpacedRectSide\",\"uuid\":\"c70de7f2-3715-43c3-9599-c736073893c8\"},{\"content\":{\"connectorIds\":[\"In2\",\"In3\"],\"side\":\"TOP\"},\"type\":\"ConnectorPlacement.EquallySpacedRectSide\",\"uuid\":\"1a48b6dd-1bbf-47fb-a945-4a4baa930d91\"},{\"content\":{\"connectorIds\":[],\"side\":\"HIDDEN\"},\"type\":\"ConnectorPlacement.EquallySpacedRectSide\",\"uuid\":\"709f434a-be22-4ab0-8c88-5861684d60a0\"}]},\"type\":\"ConnectorPlacement.EquallySpacedConnector\",\"uuid\":\"7491e8e9-2ed3-4647-a2c4-91fc44b544f7\"}],\"packageUris\":[\"http://schema.mathworks.com/mf0/Connector/R2020b\"],\"version\":\"1.0\"}"
  atan : MATLAB Function  TreatAsAtomicUnit=on
  thme_est : Outport
  wme_est : Outport  Port=2
  wires:
  iabc/1 -> Rev_Park + Rev_Clarke1/1(Iabc)
  Demux3/1 -> alpha axis observer/2(i_alpha_ref)
  Demux3/2 -> alpha axis observer2/2(i_beta_ref)
  alpha axis observer2/1(e_beta(k+1)) -> Scope/2, Discrete Filter3/1, atan/2(eq)
  atan/1(thme) -> Scope2/3, PII/1(e)
  Rate Transition2/1 -> [THME_EST], thme_est/1
  Rate Transition3/1 -> [WME_EST], wme_est/1
  PII/2(th_est) -> Scope2/2
  Rev_Park + Rev_Clarke1/1(AB) -> Demux3/1
  Classic PLL1/2(wme_est1) -> Rate Transition3/1
  Classic PLL1/1(thme_est1) -> Rate Transition2/1
  wel_meas/1 -> ?
  In6/1 -> Demux/1
  Demux/1 -> Scope3/1, alpha axis observer/1(u_alpha)
  Demux/2 -> Scope3/2, alpha axis observer2/1(u_beta)
  UA/1 -> Scope3/3
  alpha axis observer/1(e_alpha(k+1)) -> Discrete Filter1/1, Scope/1
  UB/1 -> Scope3/4
  [WME_EST] -> alpha axis observer2/3(wel_est), alpha axis observer/3(wel_est)
  Discrete Filter3/1 -> Classic PLL1/2(e_beta)
  Discrete Filter1/1 -> Classic PLL1/1(e_alpha)
